simulink library "sysgenFloatingPointFIR_Lib"  (Simulink 7.5)
settings: Solver=ode45  StartTime=0.0  StopTime=10.0  RelTol=1e-3
libraries: xbsIndex_r4 x6
settings Model: Creator=umangp  LastModifiedBy=arvinds

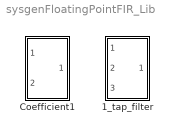
== system sysgenFloatingPointFIR_Lib ==
  1_tap_filter : Subsystem  mask{filter_coefficient=0.0356383617116066}
      mask prompts: filter_coefficient "Filter Coefficient"
  Coefficient1 : Subsystem  mask{coeff=0.0356383617116066}
      mask prompts: coeff "co_eff"

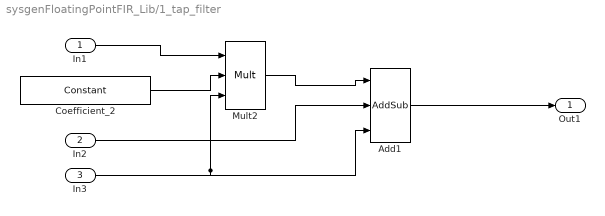
== system sysgenFloatingPointFIR_Lib/1_tap_filter ==
  In1 : Inport
  In2 : Inport  Port=2
  In3 : Inport  Port=3
  Add1 : xbsIndex_r4/AddSub  mode=Addition  use_carryin=off  use_carryout=off  en=on  latency=1  precision=Full  arith_type=Unsigned  n_bits=16  bin_pt=14  quantization=Truncate  overflow=Wrap  dbl_ovrd=off  use_behavioral_HDL=off  hw_selection=Fabric  pipelined=off  block_type=addsub
      settings: block_version=13.2
  Coefficient_2 : xbsIndex_r4/Constant  const=filter_coefficient  gui_display_data_type=Floating-point  arith_type=Floating-point  n_bits=16  bin_pt=14  preci_type=Single  exp_width=6  frac_width=15  explicit_period=off  period=1  equ=P=C  opselect=C  inp2=PCIN>>17  opr=+  inp1=P  carry=CIN  dbl_ovrd=off  block_type=constant
      settings: block_version=13.2
  Mult2 : xbsIndex_r4/Mult  precision=Full  arith_type="Signed  (2's comp)"  n_bits=16  bin_pt=14  quantization=Truncate  overflow=Wrap  en=on  latency=1  dbl_ovrd=off  use_behavioral_HDL=off  opt=Speed  use_embedded=on  optimum_pipeline=off  pipeline=on  use_rpm=on  placement_style=Triangular  block_type=mult
      settings: block_version=13.2
  Out1 : Outport
  wires:
  Coefficient_2/1 -> Mult2/2
  In2/1 -> Add1/2
  In1/1 -> Mult2/1
  Mult2/1 -> Add1/1
  Add1/1 -> Out1/1
  In3/1 -> Mult2/3, Add1/3

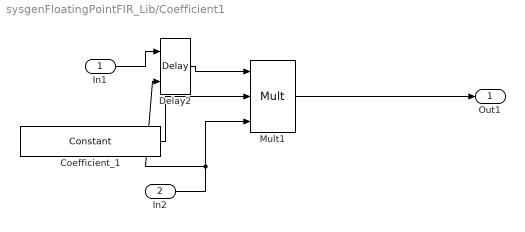
== system sysgenFloatingPointFIR_Lib/Coefficient1 ==
  In1 : Inport
  In2 : Inport  Port=2
  Coefficient_1 : xbsIndex_r4/Constant  const=coeff  gui_display_data_type=Floating-point  arith_type=Floating-point  n_bits=32  bin_pt=28  preci_type=Single  exp_width=6  frac_width=15  explicit_period=off  period=1  equ=P=C  opselect=C  inp2=PCIN>>17  opr=+  inp1=P  carry=CIN  dbl_ovrd=off  block_type=constant
      settings: block_version=13.2
  Delay2 : xbsIndex_r4/Delay  rst=off  infoeditControl=Selection of Reset will increase slice count due to use of real FFs and instead of SRLs  en=on  latency=1  dbl_ovrd=off  reg_retiming=off  block_type=delay
      settings: block_version=13.2
  Mult1 : xbsIndex_r4/Mult  precision=Full  arith_type="Signed  (2's comp)"  n_bits=16  bin_pt=14  quantization=Truncate  overflow=Wrap  en=on  latency=1  dbl_ovrd=off  use_behavioral_HDL=off  opt=Speed  use_embedded=on  optimum_pipeline=off  pipeline=on  use_rpm=on  placement_style=Triangular  block_type=mult
      settings: block_version=13.2
  Out1 : Outport
  wires:
  Delay2/1 -> Mult1/1
  In1/1 -> Delay2/1
  Mult1/1 -> Out1/1
  Coefficient_1/1 -> Mult1/2
  In2/1 -> Delay2/2, Mult1/3
